simulink model "lab4"  (R2020b)
settings: Solver=ode1  StartTime=0.0  StopTime=inf  FixedStep=0.002  RelTol=1e-3  EnableMultiTasking=on
PostLoadFcn:
  | qc_set_target_type(getConfigSet(bdroot, 'QUARC Default Target Configuration'));
values from neighbouring files (symbols this model uses):
  Ad = [1 T 0 0 0 0;0 1 0 0 0 0;0 0 1 T 0 0;0 0 0 1 0 0;1/2*K3*T*T 1/6*K3*T*T*T 0 0 1 T;K3*T 1/2*K3*T*T 0 0 0 1]    [labinithelilab4.m]
  Bd = [0 1/2*K1*T*T;0 K1*T;1/2*K2*T*T 0;K2*T 0;0 1/24*K1*K3*T*T*T*T;0 1/6*K1*K3*T*T*T]    [labinithelilab4.m]
  Cd = [1 0 0 0 0 0;0 1 0 0 0 0;0 0 1 0 0 0;0 0 0 1 0 0;0 0 0 0 0 1]    [labinithelilab4.m]
  F = importdata("flyingtimeseries.mat")    [getcovariancematrix.m]    (also in labinitheli.m = [K(1,1) K(1,3);K(2,1) K(2,3)]; labinithelilab3.m = [K(1,1) K(1,3);K(2,1) K(2,3)]; labinithelilab4.m = [K(1,1) K(1,3);K(2,1) K(2,3)])
  I = eye(6,6)    [labinithelilab4.m]
  Joystick_gain_x = 1    [labinitheli.m]    (also in labinithelilab3.m; labinithelilab4.m)
  Joystick_gain_y = -1    [labinitheli.m]    (also in labinithelilab3.m; labinithelilab4.m)
  K = lqr(A2,B2,Q,R)    [labinitheli.m]    (also in labinithelilab3.m; labinithelilab4.m)
  Qd = [5 0 0 0 0 0;0 5 0 0 0 0;0 0 5 0 0 0;0 0 0 5 0 0;0 0 0 0 5 0;0 0 0 0 0 5]    [labinithelilab4.m]
  Rd = cov(FlyData(2:6,1:6)')    [labinithelilab4.m]
undefined symbols (not defined in the file or in its folder): Discrete, HIL, qc_get_step_size, Time
libraries: quarc_library x9, ctrlSharedLib x1
settings Model: SimulationMode=external  ExtModeTrigDuration=100000  Creator=Rchan  LastModifiedBy=adamgm
settings SolverCC: PositivePriorityOrder=on
settings DataIOCC: LimitDataPoints=on  SaveFormat=Array  SignalLoggingSaveFormat=ModelDataLogs  ReturnWorkspaceOutputs=off
settings OptimizationCC: ExpressionDepthLimit=2147483647  InitFltsAndDblsToZero=on  LifeSpan=inf
settings DebuggingCC: SaveWithParameterizedLinksMsg=none  UnderspecifiedInitializationDetection=Classic  MergeDetectMultiDrivingBlocksExec=none  SolverPrmCheckMsg=warning  MultiTaskDSMMsg=warning  MultiTaskCondExecSysMsg=none  FcnCallInpInsideContextMsg=warning  AllowSymbolicDim=off  StateNameClashWarn=warning  SFUnexpectedBacktrackingDiag=warning  SFNoUnconditionalDefaultTransitionDiag=warning  SFExecutionAtInitializationDiag=none  ArithmeticOperatorsInVariantConditions=warning
settings HardwareCC: ProdBitPerPointer=32  ProdBitPerSizeT=32  ProdBitPerPtrDiffT=32  ProdLargestAtomicFloat=None  ProdIntDivRoundTo=Undefined  ProdEndianess=Unspecified  ProdWordSize=32  ProdHWDeviceType=32-bit Generic
settings ModelReferenceCC: PropagateSignalLabelsOutOfModel=off
settings SFSimCC: SimUseLocalCustomCode=off  CustomCodeUndefinedFunction=UseInterfaceOnly
settings RTWCC: Description=QUARC Win64 Target  SystemTargetFile=quarc_win64.tlc  TemplateMakefile=quarc_default_tmf  RTWUseLocalCustomCode=off
settings CodeAppCC: StateflowObjectComments=on
settings GRTTargetCC: TargetLangStandard=C89/C90 (ANSI)  ParMdlRefBuildCompliant=off  CompOptLevelCompliant=off  CombineOutputUpdateFcns=off  MatFileLogging=off  GRTInterface=on  UseToolchainInfoCompliant=off  ExtMode=on  ExtModeMexFile=quarc_comm
settings ConfigComp: CovMetricSettings=dw  CovSaveCumulativeToWorkspaceVar=on  CovSaveSingleToWorkspaceVar=on  CovExternalEMLEnable=off  CovSFcnEnable=off

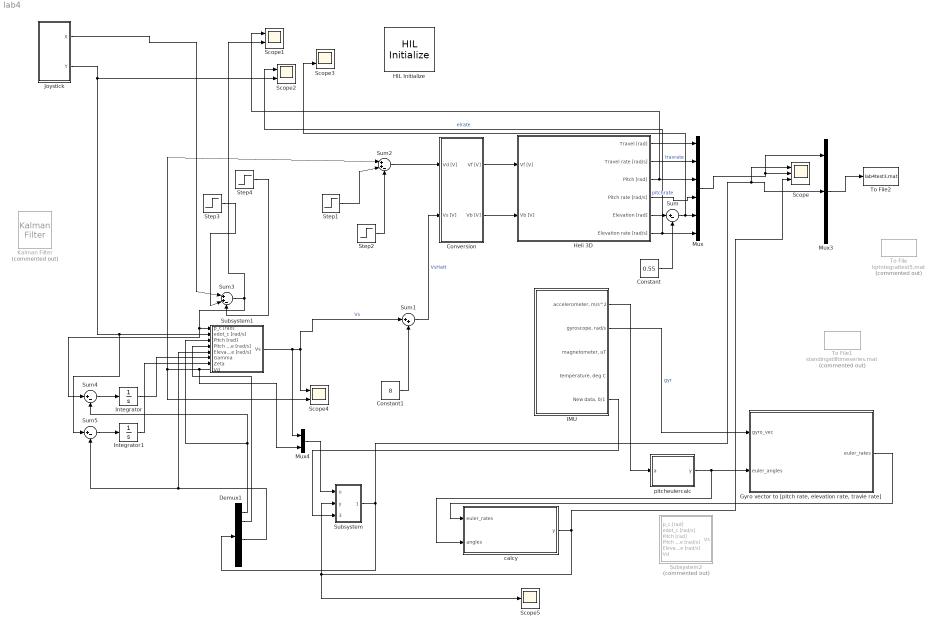
== system lab4 ==
  Constant : Constant  Value=0.55
  Constant1 : Constant  Value=8
  Conversion : Subsystem
  Demux1 : Demux  Outputs=6
  "Gyro vector to [pitch rate, elevation rate, travle rate]" : MATLAB Function  TreatAsAtomicUnit=on
  HIL Initialize : quarc_library/Data Acquisition/Generic/Configuration/HIL Initialize  Priority=-99  object_name=HIL-1  board_type=q8_usb  board_number=0  board_options=update_rate=normal;decimation=1  exclusive=off  active=off  hardware_clocks=[0:2]  clock_modes=[]  initial_clock_frequencies=[]  set_clock_params_at_start=off  set_clock_params_at_switch_in=off  set_clock_frequencies_at_start=off  set_clock_frequencies_at_switch_in=off  analog_input_channels=[0:7]  analog_input_configurations=[]  analog_input_maximums=10  analog_input_minimums=-10  set_analog_input_params_at_start=on  set_analog_input_params_at_switch_in=off  analog_output_channels=[0:7]  analog_output_maximums=10  analog_output_minimums=-10  initial_analog_outputs=[0]  final_analog_outputs=[0]  watchdog_analog_outputs=0  set_analog_output_params_at_start=on  set_analog_output_params_at_switch_in=off  set_analog_outputs_at_start=on  set_analog_outputs_at_switch_in=off  set_analog_outputs_at_terminate=on  set_analog_outputs_at_switch_out=off  set_analog_outputs_on_watchdog=off  digital_input_channels=[]  digital_output_channels=[]  digital_output_configuration=[]  initial_digital_outputs=[1]  final_digital_outputs=[1]  watchdog_digital_outputs=[1]  set_digital_output_params_at_start=off  set_digital_output_params_at_switch_in=off  set_digital_outputs_at_start=on  set_digital_outputs_at_switch_in=off  set_digital_outputs_at_terminate=on  set_digital_outputs_at_switch_out=off  set_digital_outputs_on_watchdog=off  encoder_channels=[0:7]  quadrature=[4]  encoder_filter_frequency=[]  initial_encoder_counts=[0]  set_encoder_params_at_start=on  set_encoder_params_at_switch_in=off  set_encoder_counts_at_start=on  set_encoder_counts_at_switch_in=off  pwm_channels=[0:7]  pwm_modes=0  pwm_frequency=99.532799999999995e6/4095  pwm_configuration=[0]  pwm_alignment=[0]  pwm_polarity=[1]  pwm_leading_deadband=[0]  pwm_trailing_deadband=[0]  initial_pwm_outputs=[0]  final_pwm_outputs=[0]  watchdog_pwm_outputs=[0]  set_pwm_params_at_start=on  set_pwm_params_at_switch_in=off  set_pwm_outputs_at_start=on  set_pwm_outputs_at_switch_in=off  set_pwm_outputs_at_terminate=on  set_pwm_outputs_at_switch_out=off  set_pwm_outputs_on_watchdog=off  other_output_channels=[]  initial_other_outputs=[]  final_other_outputs=[]  watchdog_other_outputs=[]  set_other_outputs_at_start=off  set_other_outputs_at_switch_in=off  set_other_outputs_at_terminate=off  set_other_outputs_at_switch_out=off  set_other_outputs_on_watchdog=off
  Heli 3D : Subsystem
  IMU : Subsystem
  Integrator : Integrator
  Integrator1 : Integrator
  Joystick : Subsystem
  Kalman Filter : ctrlSharedLib/Kalman Filter  Commented=on  TimeDomain=Discrete-Time  UseCurrentEstimator=on  ModelSource=LTI State-Space Variable  ModelSourceVariable=ss(0.95,1,1,0,1)  A=0.95  B=1  C=1  D=0  NumberOfStates=1  NumberOfInputs=1  NumberOfOutputs=1  InitialEstimateSource=Dialog  X0=0  P0=10  UseK=off  UseGH=off  NumberOfProcessNoiseInputs=1  G=1  TimeInvariantG=on  H=0  TimeInvariantH=on  Q=0.05  TimeInvariantQ=on  R=1  TimeInvariantR=on  N=0  TimeInvariantN=on  AddInputPort=on  AddEnablePort=off  OutputEstimatedY=off  OutputP=off  Ts=-1
  Mux : Mux  Inputs=6
  Mux3 : Mux  Inputs=3
  Mux4 : Mux  Inputs=2
  Scope : Scope  NumInputPorts=3
  Scope{1..4} (4 alike) : Scope  NumInputPorts=2
  Scope5 : Scope  NumInputPorts=3
  Step1 : Step  Time=13  After=0  SampleTime=0
  Step2 : Step  Time=13.2  After=0  SampleTime=0
  Step3 : Step  Time=3  After=0  SampleTime=0
  Step4 : Step  Time=8  After=0  SampleTime=0
  Subsystem : Subsystem
  Subsystem1 : Subsystem
      settings: PortSchema="{\"entries\":[{\"content\":{\"sides\":[{\"content\":{\"connectorIds\":[\"In1\",\"In2\",\"In3\",\"In4\",\"In5\",\"In6\",\"In7\",\"Out2\"]},\"type\":\"ConnectorPlacement.EquallySpacedRectSide\",\"uuid\":\"42b6e806-076b-4c56-8c54-cc10da0c9fe1\"},{\"content\":{\"connectorIds\":[\"Out1\"],\"side\":\"RIGHT\"},\"type\":\"ConnectorPlacement.EquallySpacedRectSide\",\"uuid\":\"17e06419-92a3-4202-8f3b-346b055a9ac9\"},{\"content\":{\"connectorIds\":[],\"side\":\"TOP\"},\"type\":\"ConnectorPlacement.EquallySpacedRectSide\",\"uuid\":\"184e6e7b-10a5-4c5c-94e1-4d7aed7ebe95\"},{\"content\":{\"connectorIds\":[],\"side\":\"HIDDEN\"},\"type\":\"ConnectorPlacement.EquallySpacedRectSide\",\"uuid\":\"7a97b522-4a65-499c-a7ab-0e55858670f4\"}]},\"type\":\"ConnectorPlacement.EquallySpacedConnector\",\"uuid\":\"dd461c87-29a2-471f-aec4-8ff6548faa43\"}],\"packageUris\":[\"http://schema.mathworks.com/mf0/Connector/R2020b\"],\"version\":\"1.0\"}"
  Subsystem2 : Subsystem  Commented=on
      settings: PortSchema="{\"entries\":[{\"content\":{\"sides\":[{\"content\":{\"connectorIds\":[\"In1\",\"In2\",\"In3\",\"In4\",\"In5\",\"Out2\"]},\"type\":\"ConnectorPlacement.EquallySpacedRectSide\",\"uuid\":\"42b6e806-076b-4c56-8c54-cc10da0c9fe1\"},{\"content\":{\"connectorIds\":[\"Out1\"],\"side\":\"RIGHT\"},\"type\":\"ConnectorPlacement.EquallySpacedRectSide\",\"uuid\":\"17e06419-92a3-4202-8f3b-346b055a9ac9\"},{\"content\":{\"connectorIds\":[],\"side\":\"TOP\"},\"type\":\"ConnectorPlacement.EquallySpacedRectSide\",\"uuid\":\"184e6e7b-10a5-4c5c-94e1-4d7aed7ebe95\"},{\"content\":{\"connectorIds\":[],\"side\":\"HIDDEN\"},\"type\":\"ConnectorPlacement.EquallySpacedRectSide\",\"uuid\":\"7a97b522-4a65-499c-a7ab-0e55858670f4\"}]},\"type\":\"ConnectorPlacement.EquallySpacedConnector\",\"uuid\":\"dd461c87-29a2-471f-aec4-8ff6548faa43\"}],\"packageUris\":[\"http://schema.mathworks.com/mf0/Connector/R2020b\"],\"version\":\"1.0\"}"
  Sum : Sum  Inputs=|+-
  Sum1 : Sum  Inputs=|++
  Sum2 : Sum  Inputs=|++-
  Sum3 : Sum  Inputs=|++-
  Sum4 : Sum  Inputs=|+-
  Sum5 : Sum  Inputs=|+-
  To File : ToFile  Commented=on  Filename=lqrintegraltest5.mat
  To File1 : ToFile  Commented=on  Filename=standingstilltimeseries.mat
  To File2 : ToFile  Filename=lab4test3.mat
  calcy : Subsystem
  pitcheulercalc : MATLAB Function  TreatAsAtomicUnit=on
  wires:
  Heli 3D/5(Elevation [rad]) -> Sum/1
  Mux/1 -> Mux3/1, Scope/2
  Constant/1 -> Sum/2
  Sum1/1 -> Conversion/2(Vs [V])  "VsHatt"
  Heli 3D/6(Elevation rate [rad/s]) -> Scope2/1, Mux/6  "elrate"
  Joystick/1(X) -> Sum3/1
  Joystick/2(Y) -> Sum5/1, Subsystem1/2(edot_c [rad/s]), Scope2/2
  Subsystem1/1(Vs) -> Mux4/1, Sum1/1, Scope4/1  "Vs"
  Subsystem1/2(Vd) -> Mux4/2, Sum2/1, Scope4/2
  Heli 3D/2(Travel rate [rad/s]) -> Mux/2  "travrate"
  Heli 3D/3(Pitch [rad]) -> Scope1/1, Mux/3
  Heli 3D/4(Pitch rate [rad/s]) -> Mux/4  "pitchrate"
  Sum/1 -> Scope3/2, Mux/5
  Constant1/1 -> Sum1/2
  Step1/1 -> Sum2/2
  Step2/1 -> Sum2/3
  Sum2/1 -> Conversion/1(Vd [V])
  Sum3/1 -> Scope1/2, Sum4/1, Subsystem1/1(p_c [rad])
  Step3/1 -> Sum3/2
  Step4/1 -> Sum3/3
  Sum4/1 -> Integrator/1
  Integrator/1 -> Subsystem1/6(Gamma)
  Sum5/1 -> Integrator1/1
  Integrator1/1 -> Subsystem1/7(Zeta)
  pitcheulercalc/1(y) -> calcy/2(angles), "Gyro vector to [pitch rate, elevation rate, travle rate]"/2(euler_angles)
  IMU/1("accelerometer, m/s^2") -> pitcheulercalc/1(a)
  IMU/2("gyroscope, rad/s") -> "Gyro vector to [pitch rate, elevation rate, travle rate]"/1(gyro_vec)  "gyr"
  "Gyro vector to [pitch rate, elevation rate, travle rate]"/1(euler_rates) -> calcy/1(euler_rates)
  calcy/1(y) -> Scope5/2, Subsystem/2(y), Scope/3
  Mux3/1 -> To File2/1
  Conversion/1(Vf [V]) -> Heli 3D/1(Vf [V])
  Conversion/2(Vb [V]) -> Heli 3D/2(Vb [V])
  Heli 3D/1(Travel [rad]) -> Mux/1
  Mux4/1 -> Subsystem/1(u)
  Subsystem/1(xhatt) -> Mux3/2, Scope/1, Demux1/1
  Demux1/1 -> Subsystem1/3(Pitch [rad]), Sum4/2
  Demux1/2 -> Subsystem1/4(Pitch rate [rad/s])
  Demux1/4 -> Subsystem1/5(Elevation rate [rad/s]), Sum5/2
  IMU/5("New data, 0/1") -> Subsystem/3(new_data)

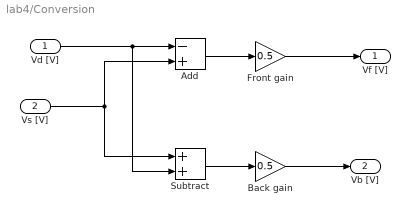
== system lab4/Conversion ==
  Vd [V] : Inport
  Vs [V] : Inport  Port=2
  Add : Sum  Inputs=-+
  Back gain : Gain  Gain=0.5
  Front gain : Gain  Gain=0.5
  Subtract : Sum
  Vf [V] : Outport
  Vb [V] : Outport  Port=2
  wires:
  Vd [V]/1 -> Subtract/2, Add/1
  Vs [V]/1 -> Subtract/1, Add/2
  Subtract/1 -> Back gain/1
  Back gain/1 -> Vb [V]/1
  Add/1 -> Front gain/1
  Front gain/1 -> Vf [V]/1

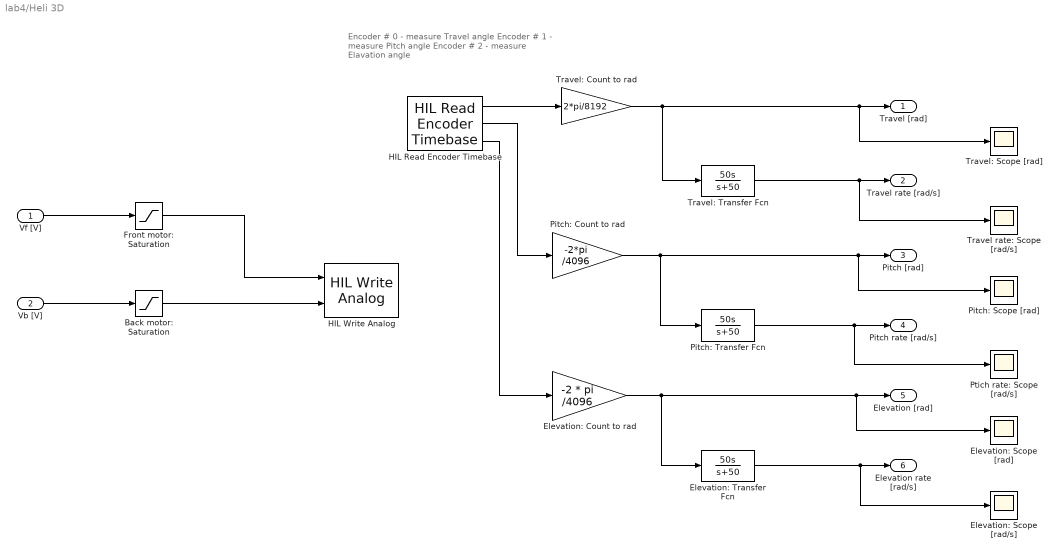
== system lab4/Heli 3D ==
  note: Encoder # 0 - measure Travel angle
      | Encoder # 1 - measure Pitch angle
      | Encoder # 2 - measure Elavation angle
  Vf [V] : Inport
  Vb [V] : Inport  Port=2
  Back motor: Saturation : Saturate  UpperLimit=5  LowerLimit=-5
  Elevation: Count to rad : Gain  Gain=-2 * pi /4096
  Elevation: Scope [rad/s] : Scope
  Elevation: Scope [rad] : Scope
  Elevation: Transfer Fcn : TransferFcn  Numerator=[50 0]  Denominator=[1 50]
  Front motor: Saturation : Saturate  UpperLimit=5  LowerLimit=-5
  HIL Read Encoder Timebase : quarc_library/Data Acquisition/Generic/Timebases/HIL Read Encoder Timebase  object_name=HIL-1  clock=0  channels=[0:2]  active=on  vector_output=off  data_type_mode=Inherit via back propagation  data_type=double  overflow_mode=Error on overflow  samples_in_buffer=max(ceil(1/qc_get_step_size), 1)
  HIL Write Analog : quarc_library/Data Acquisition/Generic/Immediate I//O/HIL Write Analog  object_name=HIL-1  channels=[0:1]  sample_time=-1  active=off  vector_input=off
  Pitch: Count to rad : Gain  Gain=-2*pi /4096
  Pitch: Scope [rad] : Scope
  Pitch: Transfer Fcn : TransferFcn  Numerator=[50 0]  Denominator=[1 50]
  Ptich rate: Scope [rad/s] : Scope
  Travel rate: Scope [rad/s] : Scope
  Travel: Count to rad : Gain  Gain=2*pi/8192
  Travel: Scope [rad] : Scope
  Travel: Transfer Fcn : TransferFcn  Numerator=[50 0]  Denominator=[1 50]
  Travel [rad] : Outport
  Travel rate [rad/s] : Outport  Port=2
  Pitch [rad] : Outport  Port=3
  Pitch rate [rad/s] : Outport  Port=4
  Elevation [rad] : Outport  Port=5
  Elevation rate [rad/s] : Outport  Port=6
  wires:
  HIL Read Encoder Timebase/1 -> Travel: Count to rad/1
  HIL Read Encoder Timebase/2 -> Pitch: Count to rad/1
  HIL Read Encoder Timebase/3 -> Elevation: Count to rad/1
  Travel: Count to rad/1 -> Travel: Scope [rad]/1, Travel [rad]/1, Travel: Transfer Fcn/1
  Travel: Transfer Fcn/1 -> Travel rate: Scope [rad/s]/1, Travel rate [rad/s]/1
  Pitch: Count to rad/1 -> Pitch: Transfer Fcn/1, Pitch: Scope [rad]/1, Pitch [rad]/1
  Pitch: Transfer Fcn/1 -> Ptich rate: Scope [rad/s]/1, Pitch rate [rad/s]/1
  Elevation: Count to rad/1 -> Elevation: Transfer Fcn/1, Elevation: Scope [rad]/1, Elevation [rad]/1
  Elevation: Transfer Fcn/1 -> Elevation: Scope [rad/s]/1, Elevation rate [rad/s]/1
  Vf [V]/1 -> Front motor: Saturation/1
  Vb [V]/1 -> Back motor: Saturation/1
  Front motor: Saturation/1 -> HIL Write Analog/1
  Back motor: Saturation/1 -> HIL Write Analog/2

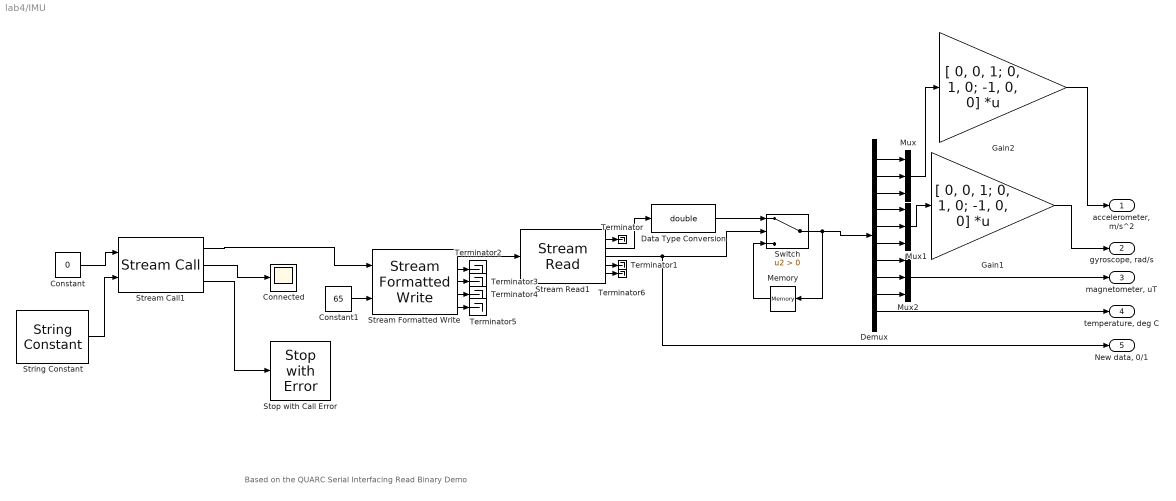
== system lab4/IMU ==
  note: Based on the QUARC Serial Interfacing Read Binary Demo
  Connected : Scope
  Constant : Constant  Value=0
  Constant1 : Constant  Value=65
  Data Type Conversion : DataTypeConversion  OutDataTypeStr=double
  Demux : Demux  Outputs=10
  Gain1 : Gain  Gain=[ 0, 0, 1; 0, 1, 0; -1, 0, 0]  Multiplication=Matrix(K*u) (u vector)
  Gain2 : Gain  Gain=[ 0, 0, 1; 0, 1, 0; -1, 0, 0]  Multiplication=Matrix(K*u) (u vector)
  Memory : Memory  InitialCondition=[0 0 0 0 0 0 0 0 0 0]
  Mux : Mux  Inputs=3
  Mux1 : Mux  Inputs=3
  Mux2 : Mux  Inputs=3
  Stop with Call Error : quarc_library/Sinks/Error Handling/Stop with Error  message_type=Interpret input as error code  message=Error occurred
      settings: SourceProductName=QUARC Targets
  Stream Call1 : quarc_library/Communications/Intermediate/Stream Call  uri_source=External input port  uri=serial://IMU:9?baud=115200,word=8,parity=none,stop=1,flow='none'  apply_uri_to_all_configs=on  send_buffer_size=8000  receive_buffer_size=8000  byte_order=little endian (Intel - LSB first)  sample_time=qc_get_step_size  non_blocking=on  active=off
      settings: SourceProductName=QUARC Targets
  Stream Formatted Write : quarc_library/Communications/Intermediate/Stream Formatted Write  format_string=%c\n  max_code_units=80  optimization=Minimizing latency
      settings: SourceProductName=QUARC Targets
  Stream Read1 : quarc_library/Communications/Intermediate/Stream Read  data_type=single  type_expr=BusObject  num_elements=10  receive_dims=off
      settings: SourceProductName=QUARC Targets
  String Constant : quarc_library/Strings/String Constant  string_value=qc_perform_substitutions('serial://IMU:%{PORT}?baud=115200,word=8,parity=none,stop=1')  evaluate_string=on  string_type=URI  max_length=255  sample_time=inf  variable_size=off
      settings: AttributesFormatString="\"serial://IMU:5?baud=115200,word=8,parity=none,stop=1\""  SourceProductName=QUARC Targets
  Switch : Switch  Criteria=u2 > Threshold
  Terminator{,1..6} (7 alike) : Terminator
  "accelerometer, m/s^2" : Outport
  "gyroscope, rad/s" : Outport  Port=2
  "magnetometer, uT" : Outport  Port=3
  "temperature, deg C" : Outport  Port=4
  "New data, 0/1" : Outport  Port=5
  wires:
  Switch/1 -> Memory/1, Demux/1
  Data Type Conversion/1 -> Switch/1
  Stream Read1/3 -> "New data, 0/1"/1, Switch/2
  Stream Formatted Write/1 -> Stream Read1/1
  Constant1/1 -> Stream Formatted Write/2
  Gain1/1 -> "gyroscope, rad/s"/1
  Gain2/1 -> "accelerometer, m/s^2"/1
  Stream Read1/4 -> Terminator1/1
  Demux/10 -> "temperature, deg C"/1
  Mux1/1 -> Gain1/1
  Stream Read1/2 -> Data Type Conversion/1
  Demux/7 -> Mux2/1
  Demux/8 -> Mux2/2
  Demux/9 -> Mux2/3
  Mux2/1 -> "magnetometer, uT"/1
  Demux/6 -> Mux1/3
  Demux/5 -> Mux1/2
  Demux/4 -> Mux1/1
  Mux/1 -> Gain2/1
  Demux/3 -> Mux/3
  Demux/1 -> Mux/1
  Demux/2 -> Mux/2
  Stream Read1/1 -> Terminator/1
  Stream Call1/1 -> Stream Formatted Write/1
  Constant/1 -> Stream Call1/1
  String Constant/1 -> Stream Call1/2
  Stream Call1/2 -> Connected/1
  Stream Call1/3 -> Stop with Call Error/1
  Memory/1 -> Switch/3
  Stream Formatted Write/2 -> Terminator2/1
  Stream Formatted Write/3 -> Terminator3/1
  Stream Formatted Write/4 -> Terminator4/1
  Stream Formatted Write/5 -> Terminator5/1
  Stream Read1/5 -> Terminator6/1

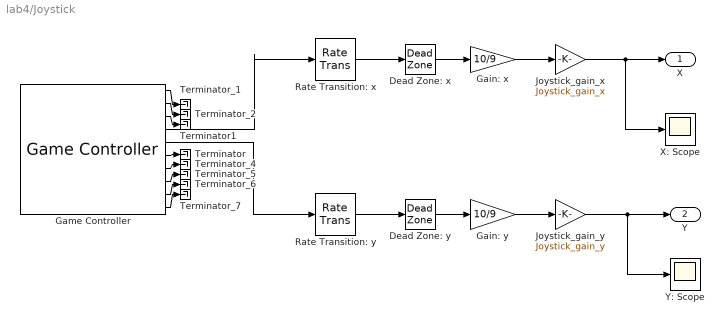
== system lab4/Joystick ==
  Dead Zone: x : DeadZone  LowerValue=-0.1  UpperValue=0.1  SaturateOnIntegerOverflow=on
  Dead Zone: y : DeadZone  LowerValue=-0.1  UpperValue=0.1  SaturateOnIntegerOverflow=on
  Gain: x : Gain  Gain=10/9
  Gain: y : Gain  Gain=10/9
  Game Controller : quarc_library/Devices/Peripherals/Target/Game Controller  controller=1  buffer_size=12  deadzone=[]  saturation=[]  sample_time=max(qc_get_step_size, 0.01)  auto_center=off  enabled=on
      settings: SourceProductName=QUARC Targets
  Joystick_gain_x : Gain  Gain=Joystick_gain_x
  Joystick_gain_y : Gain  Gain=Joystick_gain_y
  Rate Transition: x : RateTransition
  Rate Transition: y : RateTransition
  Terminator : Terminator
  Terminator1 : Terminator
  Terminator_{1..2,4..7} (6 alike) : Terminator
  X: Scope : Scope
  Y: Scope : Scope
  X : Outport
  Y : Outport  Port=2
  wires:
  Rate Transition: y/1 -> Dead Zone: y/1
  Rate Transition: x/1 -> Dead Zone: x/1
  Game Controller/5 -> Rate Transition: y/1
  Game Controller/4 -> Rate Transition: x/1
  Game Controller/1 -> Terminator_1/1
  Game Controller/2 -> Terminator_2/1
  Game Controller/7 -> Terminator_4/1
  Game Controller/8 -> Terminator_5/1
  Game Controller/9 -> Terminator_6/1
  Game Controller/10 -> Terminator_7/1
  Game Controller/3 -> Terminator1/1
  Game Controller/6 -> Terminator/1
  Dead Zone: x/1 -> Gain: x/1
  Dead Zone: y/1 -> Gain: y/1
  Gain: x/1 -> Joystick_gain_x/1
  Gain: y/1 -> Joystick_gain_y/1
  Joystick_gain_x/1 -> X/1, X: Scope/1
  Joystick_gain_y/1 -> Y: Scope/1, Y/1

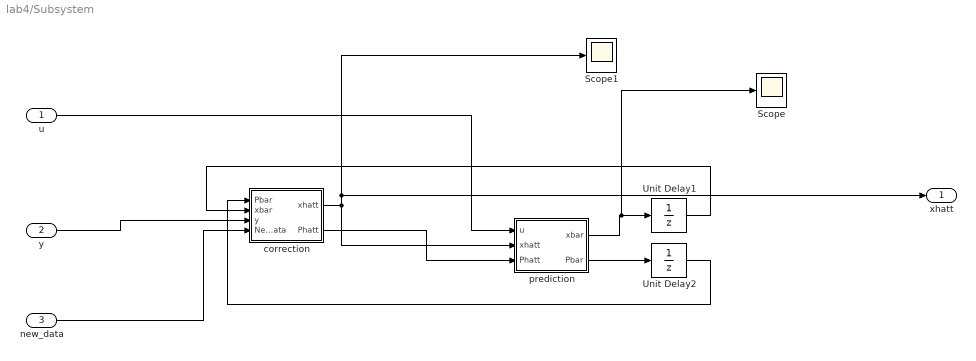
== system lab4/Subsystem ==
  u : Inport
  y : Inport  Port=2
  new_data : Inport  Port=3
  Scope : Scope
  Scope1 : Scope
  Unit Delay1 : UnitDelay  InitialCondition=[0;0;0;0;0;0]  SampleTime=-1  HasFrameUpgradeWarning=on
  Unit Delay2 : UnitDelay  InitialCondition=eye(6,6)  SampleTime=-1  HasFrameUpgradeWarning=on
  correction : MATLAB Function  TreatAsAtomicUnit=on
  prediction : MATLAB Function  TreatAsAtomicUnit=on
  xhatt : Outport
  wires:
  u/1 -> prediction/1(u)
  y/1 -> correction/3(y)
  correction/2(Phatt) -> prediction/3(Phatt)
  correction/1(xhatt) -> Scope1/1, xhatt/1, prediction/2(xhatt)
  prediction/1(xbar) -> Scope/1, Unit Delay1/1
  prediction/2(Pbar) -> Unit Delay2/1
  Unit Delay2/1 -> correction/1(Pbar)
  Unit Delay1/1 -> correction/2(xbar)
  new_data/1 -> correction/4(New_data)

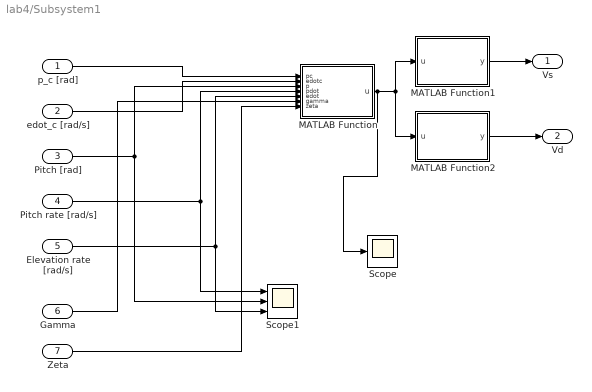
== system lab4/Subsystem1 ==
  p_c [rad] : Inport
  edot_c [rad/s] : Inport  Port=2
  Pitch [rad] : Inport  Port=3
  Pitch rate [rad/s] : Inport  Port=4
  Elevation rate [rad/s] : Inport  Port=5
  Gamma : Inport  Port=6
  Zeta : Inport  Port=7
  MATLAB Function : MATLAB Function  TreatAsAtomicUnit=on
  MATLAB Function1 : MATLAB Function  TreatAsAtomicUnit=on
  MATLAB Function2 : MATLAB Function  TreatAsAtomicUnit=on
  Scope : Scope
  Scope1 : Scope  NumInputPorts=3
  Vs : Outport
  Vd : Outport  Port=2
  wires:
  p_c [rad]/1 -> MATLAB Function/1(pc)
  Pitch [rad]/1 -> Scope1/2, MATLAB Function/3(p)
  Pitch rate [rad/s]/1 -> Scope1/1, MATLAB Function/4(pdot)
  Elevation rate [rad/s]/1 -> Scope1/3, MATLAB Function/5(edot)
  MATLAB Function/1(u) -> Scope/1, MATLAB Function1/1(u), MATLAB Function2/1(u)
  MATLAB Function1/1(y) -> Vs/1
  MATLAB Function2/1(y) -> Vd/1
  edot_c [rad/s]/1 -> MATLAB Function/2(edotc)
  Gamma/1 -> MATLAB Function/6(gamma)
  Zeta/1 -> MATLAB Function/7(zeta)

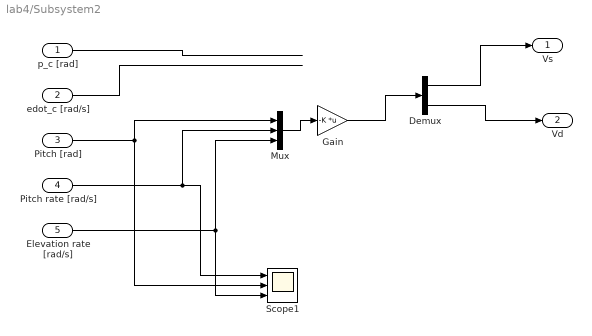
== system lab4/Subsystem2 ==
  p_c [rad] : Inport
  edot_c [rad/s] : Inport  Port=2
  Pitch [rad] : Inport  Port=3
  Pitch rate [rad/s] : Inport  Port=4
  Elevation rate [rad/s] : Inport  Port=5
  Demux : Demux  Outputs=2
  Gain : Gain  Gain=-K  Multiplication=Matrix(K*u)
  Mux : Mux  Inputs=3
  Scope1 : Scope  NumInputPorts=3
  Vs : Outport
  Vd : Outport  Port=2
  wires:
  p_c [rad]/1 -> ?
  Pitch [rad]/1 -> Mux/1, Scope1/2
  Pitch rate [rad/s]/1 -> Mux/2, Scope1/1
  Elevation rate [rad/s]/1 -> Mux/3, Scope1/3
  Demux/1 -> Vs/1
  Demux/2 -> Vd/1
  edot_c [rad/s]/1 -> ?
  Mux/1 -> Gain/1
  Gain/1 -> Demux/1

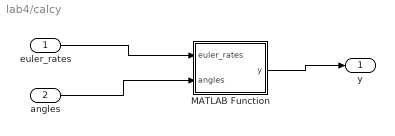
== system lab4/calcy ==
  euler_rates : Inport
  angles : Inport  Port=2
  MATLAB Function : MATLAB Function  TreatAsAtomicUnit=on
  y : Outport
  wires:
  euler_rates/1 -> MATLAB Function/1(euler_rates)
  MATLAB Function/1(y) -> y/1
  angles/1 -> MATLAB Function/2(angles)

== matlab function lab4/pitcheulercalc ==
  data: a input; y output size=[2 1]
function y = fcn(a)
ax = a(1);
ay = a(2);
az = a(3);
y = [mod(atan2(ay,az),2*pi)-pi;atan2(ax,(sqrt(ay^2+az^2)))];
end

== matlab function lab4/Gyro vector to [pitch rate, elevation rate, travle rate] ==
  data: gyro_vec input; euler_rates output; euler_angles input
function euler_rates = gyro_vec_to_euler_rates(gyro_vec,euler_angles)
%#codegen
    phi = euler_angles(1);
    theta = euler_angles(2);


    T = [1, sin(phi)*tan(theta), cos(phi)*tan(theta);
         0, cos(phi),            -sin(phi);
         0, sin(phi)/cos(theta), cos(phi)/cos(theta)]; 
euler_rates = T*gyro_vec;

== matlab function lab4/Subsystem1/MATLAB Function ==
  data: pc input; u output size=[2 1]; edotc input; p input; pdot input; edot input; gamma input; zeta input; F parameter size=[2 2]; K parameter size=[2 5]
function u = fcn(pc, edotc, p, pdot, edot,gamma,zeta,F, K)

u = F*[pc;edotc]-K*[p;pdot;edot;gamma;zeta];

end

== matlab function lab4/Subsystem1/MATLAB Function1 ==
  data: u input; y output size=[1 1]
function y = fcn(u)

y = u(1);
end

== matlab function lab4/Subsystem1/MATLAB Function2 ==
  data: u input; y output size=[1 1]
function y = fcn(u)

y = u(2);
end

== matlab function lab4/calcy/MATLAB Function ==
  data: euler_rates input; y output; angles input; Chatt parameter
function y = fcn(euler_rates,angles, Chatt)
e = angles(2);
edot = euler_rates(2);
p = angles(1);
pdot = euler_rates(1);
lamb = 0;
lambdot = euler_rates(3);
y = Chatt*[p;pdot;e;edot;lamb;lambdot];

== matlab function lab4/Subsystem/correction ==
  data: Pbar input size=[6 6]; xbar input size=[6 1]; y input; xhatt output size=[6 1]; Cd parameter; Phatt output size=[6 6]; Rd parameter; I parameter; New_data input
function [xhatt,Phatt] = fcn(Pbar,xbar,y,Cd,Rd, I, New_data)
    if New_data~=0
        L = Pbar*Cd'*inv(Cd*Pbar*Cd'+Rd);
        xhatt = xbar + L*(y-Cd*xbar);
        Phatt = (I-L*Cd)*Pbar*(I-L*Cd)'+L*Rd*L';
    else
        xhatt = xbar;
        Phatt = Pbar;
    end
end

== matlab function lab4/Subsystem/prediction ==
  data: u input; xbar output size=[6 1]; xhatt input size=[6 1]; Phatt input size=[6 6]; Pbar output size=[6 6]; Ad parameter; Bd parameter; Qd parameter
function [xbar,Pbar] = fcn(u,xhatt, Phatt,Ad, Bd, Qd)

xbar = Ad*xhatt + Bd*u;
Pbar = Ad*Phatt*Ad' + Qd;
